simulink model "foc_blcd"  (R2022a)
settings: Solver=VariableStepAuto  StartTime=0.0  StopTime=1  RelTol=1e-3
values from neighbouring files (symbols this model uses):
  Idtarget = 0    [targetinitcoeffvalues.mat]
  Iqtarget = 10    [targetinitcoeffvalues.mat]
undefined symbols (not defined in the file or in its folder): deadTime_inv, f_spin
libraries: simulink x6, spsIdealSwitchLib x6, spsSeriesRLCBranchLib x4, spsMultimeterLib x3, slpidlib x2, spsAlphaBetaZerotoabcLib x1, spsAlphaBetaZerotodq0Lib x1, spsabctoAlphaBetaZeroLib x1, spsdq0toAlphaBetaZeroLib x1, spsDCVoltageSourceLib x1, spsGroundLib x1, spspowerguiLib x1
settings Model: Creator=1  LastModifiedBy=1
settings DebuggingCC: UnderSpecifiedDimensionMsg=warning

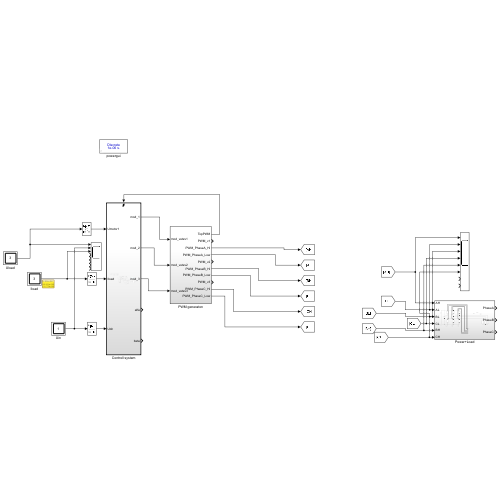
[thumbnail: Simulink's stored preview of the top-level diagram]
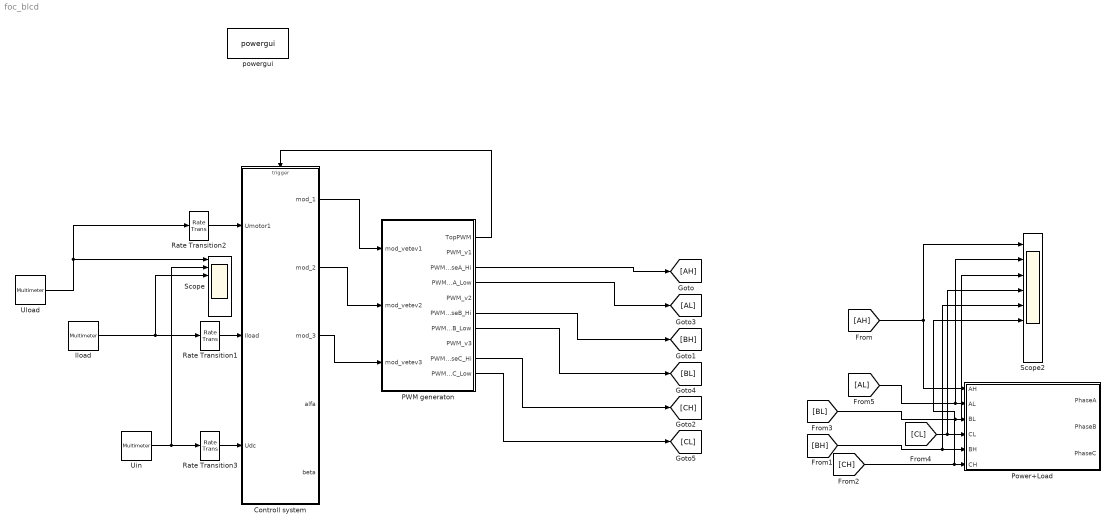
== system foc_blcd ==
  Controll system : Subsystem
  Iload : spsMultimeterLib/Multimeter  L=9  sel=[7 8 9]  yselected={}  Gain=[1 1 1]  OutputType=Complex  PlotAtSimulationStop=off  PhasorSimulation=off
  PWM generaton : Subsystem
  Power+Load : Subsystem
  Rate Transition1 : RateTransition  Integrity=off
  Rate Transition2 : RateTransition  Integrity=off
  Rate Transition3 : RateTransition  Integrity=off
  Scope : Scope  NumInputPorts=8
  Scope2 : Scope  NumInputPorts=8
  Uin : spsMultimeterLib/Multimeter  L=9  sel=1  yselected={}  Gain=1  OutputType=Complex  PlotAtSimulationStop=off  PhasorSimulation=off
  Uload : spsMultimeterLib/Multimeter  L=9  sel=[2 3 4]  yselected={}  Gain=[1 1 1]  OutputType=Complex  PlotAtSimulationStop=off  PhasorSimulation=off
  powergui : spspowerguiLib/powergui  Priority=1  SimulationMode=Discrete  SampleTime=1e-6  frequency=60  Iterations=50  frequencyindice=0  Pbase=100e6  ErrMax=1e-4  UnitsV=kV  UnitsW=MW  buscounter=0  FunctionMessages=off  echomessages=off  EnableUseOfTLC=off  CurrentSourceSwitches=off  DisableSnubberDevices=off  DisableRonSwitches=off  DisableVfSwitches=off  DisplayEquations=off  AutomaticDiscreteSolvers=off  SolverType=Tustin/Backward Euler (TBE)  Interpol=off  ExternalGateDelay=off  methode=off  Ts=100  x0status=blocks  SPID=on  SwTol=0  HookPort=off  NonlinearTolerance=1e-4  nMaxIteration=100  ContinueOnMaxIteration=off  RestoreLinks=warning  ResistiveCurrentMeasurement=off  Frange=[0:2:500]  Ylog=off  Xlog=on  ShowGrid=off  save=off  variable=ZData  structure=0  ZoomFFT=off  StartTime=0.0  cycles=1  DisplayStyle=1  fundamental=60  FreqAxis=off  MaxFrequency=1000  frequencyindicesteady=1  RmsSteady=1  display=off
  wires:
  Controll system/1(mod_1) -> PWM generaton/1(mod_vetev1)
  Controll system/2(mod_2) -> PWM generaton/2(mod_vetev2)
  Controll system/3(mod_3) -> PWM generaton/3(mod_vetev3)
  PWM generaton/1(TopPWM) -> Controll system/Trigger
  Uload/1 -> Rate Transition2/1, Scope/1
  Uin/1 -> Scope/2, Rate Transition3/1
  [AH] -> Scope2/1, Power+Load/1(AH)
  [CH] -> Scope2/6, Power+Load/6(CH)
  [BH] -> Power+Load/5(BH), Scope2/5
  [BL] -> Scope2/3, Power+Load/3(BL)
  [CL] -> Scope2/4, Power+Load/4(CL)
  [AL] -> Scope2/2, Power+Load/2(AL)
  PWM generaton/3(PWM_PhaseA_Hi) -> [AH]
  PWM generaton/4(PWM_PhaseA_Low) -> [AL]
  PWM generaton/6(PWM_PhaseB_Hi) -> [BH]
  PWM generaton/7(PWM_PhaseB_Low) -> [BL]
  PWM generaton/10(PWM_PhaseC_Low) -> [CL]
  PWM generaton/9(PWM_PhaseC_Hi) -> [CH]
  Iload/1 -> Scope/3, Rate Transition1/1
  Rate Transition2/1 -> Controll system/1(Umotor1)
  Rate Transition1/1 -> Controll system/2(Iload)
  Rate Transition3/1 -> Controll system/3(Udc)

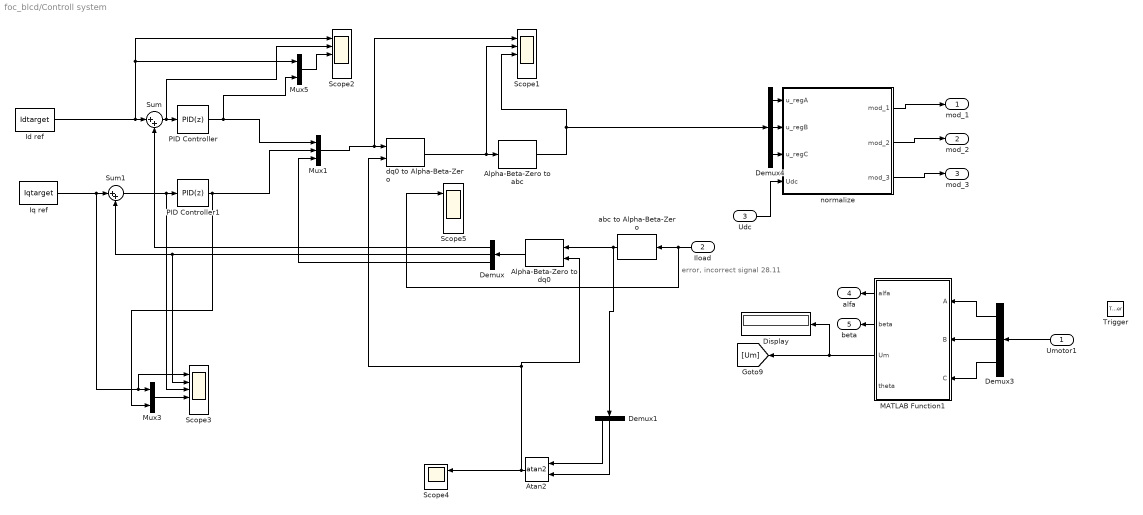
== system foc_blcd/Controll system ==
  note: error, incorrect signal 28.11
  Umotor1 : Inport
  Iload : Inport  Port=2
  Udc : Inport  Port=3
  Trigger : TriggerPort  VariantControl=(inherit)  PortDimensions=1
  Alpha-Beta-Zero to abc : spsAlphaBetaZerotoabcLib/Alpha-Beta-Zero to abc
      settings: SourceProductBaseCode=PS
  Alpha-Beta-Zero to dq0 : spsAlphaBetaZerotodq0Lib/Alpha-Beta-Zero to dq0  Alignment=90 degrees behind phase A axis
      settings: SourceProductBaseCode=PS
  Atan2 : Trigonometry  Operator=atan2
  Demux{,1,3..4} (4 alike) : Demux  Outputs=3
  Display : Display
  Id ref : Constant  Value=Idtarget
  Iq ref : Constant  Value=Iqtarget
  MATLAB Function1 : MATLAB Function  TreatAsAtomicUnit=on
  Mux1 : Mux  Inputs=3
  Mux3 : Mux  Inputs=2
  Mux5 : Mux  Inputs=2
  PID Controller : slpidlib/PID Controller  Controller=PID  Form=Parallel  TimeDomain=Discrete-time  UseExternalTs=off  SampleTime=-1  IntegratorMethod=Forward Euler  FilterMethod=Forward Euler  ControllerParametersSource=internal  P=1  I=0  UseKiTs=off  D=0  N=100  UseFilter=on  TunerSelectOption=Transfer Function Based (PID Tuner App)  InitialConditionSource=internal  InitialConditionForIntegrator=0  InitialConditionForFilter=0  DifferentiatorICPrevScaledInput=0  ExternalReset=none  TrackingMode=off  Kt=1  LimitOutput=off  SatLimitsSource=internal  UpperSaturationLimit=inf  LowerSaturationLimit=-inf  LinearizeAsGain=on  AntiWindupMode=none  Kb=1  POutMin=[]  POutMax=[]  IOutMin=[]  IOutMax=[]  DOutMin=[]  DOutMax=[]  NOutMin=[]  NOutMax=[]  SumOutMin=[]  SumOutMax=[]  SaturationOutMin=[]  SaturationOutMax=[]  PParamMin=[]  PParamMax=[]  IParamMin=[]  IParamMax=[]  DParamMin=[]  DParamMax=[]  NParamMin=[]  NParamMax=[]  KbParamMin=[]  KbParamMax=[]  KtParamMin=[]  KtParamMax=[]  KbOutMin=[]  KbOutMax=[]  KtOutMin=[]  KtOutMax=[]  IntegratorOutMin=[]  IntegratorOutMax=[]  FilterOutMin=[]  FilterOutMax=[]  SumI1OutMin=[]  SumI1OutMax=[]  SumI2OutMin=[]  SumI2OutMax=[]  SumI3OutMin=[]  SumI3OutMax=[]  SumI4OutMin=[]  SumI4OutMax=[]  SumDOutMin=[]  SumDOutMax=[]  DifferentiatorOutMin=[]  DifferentiatorOutMax=[]  FilterDiffOutCoefMin=[]  FilterDiffOutCoefMax=[]  ReciprocalOutMin=[]  ReciprocalOutMax=[]  SumDenOutMin=[]  SumDenOutMax=[]  SumNumOutMin=[]  SumNumOutMax=[]  DivideOutMin=[]  DivideOutMax=[]  UdiffTsProdOutMin=[]  UdiffTsProdOutMax=[]  NTsProdOutMin=[]  NTsProdOutMax=[]  UintegralTsProdOutMin=[]  UintegralTsProdOutMax=[]  UngainTsProdOutMin=[]  UngainTsProdOutMax=[]  IntegratorContinuousStateAttributes=''  IntegratorStateMustResolveToSignalObject=off  IntegratorRTWStateStorageClass=Auto  FilterContinuousStateAttributes=''  FilterStateMustResolveToSignalObject=off  FilterRTWStateStorageClass=Auto  ParallelPVariant=InternalParameters  IdealPVariant=Disabled  IVariant=InternalParameters  DVariant=InternalParameters  IntegratorVariant=Discrete  SatVariant=Disabled  AWVariant=Passthrough  PCopyVariant=Disabled  TRVariant=Disabled  FdbkBlocksVariant=Forward  IdealPFdbkVariant=Disabled  SatFdbkVariant=Disabled  DerivativeFilterVariant=ForwardEulerFilter  NVariant=InternalParameters  NCopyVariant=Disabled  FilterICVariant=InternalICsFilter  IntegratorICVariant=InternalICs  ExternalResetVariant=Disabled  TRSumVariant=Passthrough  SumFdbkVariant=Disabled  SumVariant=Sum_PID  TsampFilterVariant=InternalTs  TsampNgainVariant=Passthrough  TsampIntegralVariant=Passthrough  ExternalSaturationOutDataTypeStr=Inherit: Same as second input  aMode=0
  PID Controller1 : slpidlib/PID Controller  Controller=PID  Form=Parallel  TimeDomain=Discrete-time  UseExternalTs=off  SampleTime=-1  IntegratorMethod=Forward Euler  FilterMethod=Forward Euler  ControllerParametersSource=internal  P=1  I=0  UseKiTs=off  D=0  N=100  UseFilter=on  TunerSelectOption=Transfer Function Based (PID Tuner App)  InitialConditionSource=internal  InitialConditionForIntegrator=0  InitialConditionForFilter=0  DifferentiatorICPrevScaledInput=0  ExternalReset=none  TrackingMode=off  Kt=1  LimitOutput=off  SatLimitsSource=internal  UpperSaturationLimit=inf  LowerSaturationLimit=-inf  LinearizeAsGain=on  AntiWindupMode=none  Kb=1  POutMin=[]  POutMax=[]  IOutMin=[]  IOutMax=[]  DOutMin=[]  DOutMax=[]  NOutMin=[]  NOutMax=[]  SumOutMin=[]  SumOutMax=[]  SaturationOutMin=[]  SaturationOutMax=[]  PParamMin=[]  PParamMax=[]  IParamMin=[]  IParamMax=[]  DParamMin=[]  DParamMax=[]  NParamMin=[]  NParamMax=[]  KbParamMin=[]  KbParamMax=[]  KtParamMin=[]  KtParamMax=[]  KbOutMin=[]  KbOutMax=[]  KtOutMin=[]  KtOutMax=[]  IntegratorOutMin=[]  IntegratorOutMax=[]  FilterOutMin=[]  FilterOutMax=[]  SumI1OutMin=[]  SumI1OutMax=[]  SumI2OutMin=[]  SumI2OutMax=[]  SumI3OutMin=[]  SumI3OutMax=[]  SumI4OutMin=[]  SumI4OutMax=[]  SumDOutMin=[]  SumDOutMax=[]  DifferentiatorOutMin=[]  DifferentiatorOutMax=[]  FilterDiffOutCoefMin=[]  FilterDiffOutCoefMax=[]  ReciprocalOutMin=[]  ReciprocalOutMax=[]  SumDenOutMin=[]  SumDenOutMax=[]  SumNumOutMin=[]  SumNumOutMax=[]  DivideOutMin=[]  DivideOutMax=[]  UdiffTsProdOutMin=[]  UdiffTsProdOutMax=[]  NTsProdOutMin=[]  NTsProdOutMax=[]  UintegralTsProdOutMin=[]  UintegralTsProdOutMax=[]  UngainTsProdOutMin=[]  UngainTsProdOutMax=[]  IntegratorContinuousStateAttributes=''  IntegratorStateMustResolveToSignalObject=off  IntegratorRTWStateStorageClass=Auto  FilterContinuousStateAttributes=''  FilterStateMustResolveToSignalObject=off  FilterRTWStateStorageClass=Auto  ParallelPVariant=InternalParameters  IdealPVariant=Disabled  IVariant=InternalParameters  DVariant=InternalParameters  IntegratorVariant=Discrete  SatVariant=Disabled  AWVariant=Passthrough  PCopyVariant=Disabled  TRVariant=Disabled  FdbkBlocksVariant=Forward  IdealPFdbkVariant=Disabled  SatFdbkVariant=Disabled  DerivativeFilterVariant=ForwardEulerFilter  NVariant=InternalParameters  NCopyVariant=Disabled  FilterICVariant=InternalICsFilter  IntegratorICVariant=InternalICs  ExternalResetVariant=Disabled  TRSumVariant=Passthrough  SumFdbkVariant=Disabled  SumVariant=Sum_PID  TsampFilterVariant=InternalTs  TsampNgainVariant=Passthrough  TsampIntegralVariant=Passthrough  ExternalSaturationOutDataTypeStr=Inherit: Same as second input  aMode=0
  Scope{1..3,5} (4 alike) : Scope  NumInputPorts=5
  Scope4 : Scope  NumInputPorts=2
  Sum : Sum  Inputs=|++
  Sum1 : Sum  Inputs=|++
  abc to Alpha-Beta-Zero : spsabctoAlphaBetaZeroLib/abc to Alpha-Beta-Zero
      settings: SourceProductBaseCode=PS
  dq0 to Alpha-Beta-Zero : spsdq0toAlphaBetaZeroLib/dq0 to Alpha-Beta-Zero  Alignment=90 degrees behind phase A axis
      settings: SourceProductBaseCode=PS
  normalize : MATLAB Function  TreatAsAtomicUnit=on
  mod_1 : Outport
  mod_2 : Outport  Port=2
  mod_3 : Outport  Port=3
  alfa : Outport  Port=4
  beta : Outport  Port=5
  wires:
  abc to Alpha-Beta-Zero/1 -> Demux1/1, Alpha-Beta-Zero to dq0/1
  Demux4/3 -> normalize/3(u_regC)
  Id ref/1 -> Mux5/1, Scope2/1, Sum/1
  MATLAB Function1/3(Um) -> [Um], Display/1
  Demux/1 -> Sum/2
  Sum1/1 -> Scope3/3, PID Controller1/1
  Alpha-Beta-Zero to abc/1 -> Scope1/3, Demux4/1
  Mux1/1 -> Scope1/1, dq0 to Alpha-Beta-Zero/1
  Demux/2 -> Sum1/2, Scope3/2
  Demux4/1 -> normalize/1(u_regA)
  Iq ref/1 -> Scope3/1, Mux3/1, Sum1/1
  dq0 to Alpha-Beta-Zero/1 -> Scope1/2, Alpha-Beta-Zero to abc/1
  Sum/1 -> Scope2/2, PID Controller/1
  Demux3/1 -> MATLAB Function1/1(A)
  Demux/3 -> Mux1/3
  PID Controller/1 -> Mux1/1, Mux5/2
  Demux4/2 -> normalize/2(u_regB)
  Alpha-Beta-Zero to dq0/1 -> Demux/1
  PID Controller1/1 -> Mux1/2, Mux3/2
  Demux3/3 -> MATLAB Function1/3(C)
  Demux3/2 -> MATLAB Function1/2(B)
  normalize/2(mod_2) -> mod_2/1
  MATLAB Function1/2(beta) -> beta/1
  MATLAB Function1/1(alfa) -> alfa/1
  normalize/3(mod_3) -> mod_3/1
  normalize/1(mod_1) -> mod_1/1
  Umotor1/1 -> Demux3/1
  Iload/1 -> abc to Alpha-Beta-Zero/1, Scope5/1
  Udc/1 -> normalize/4(Udc)
  Atan2/1 -> Alpha-Beta-Zero to dq0/2, dq0 to Alpha-Beta-Zero/2, Scope4/1
  Demux1/1 -> Atan2/1
  Demux1/2 -> Atan2/2
  Mux3/1 -> Scope3/4
  Mux5/1 -> Scope2/3

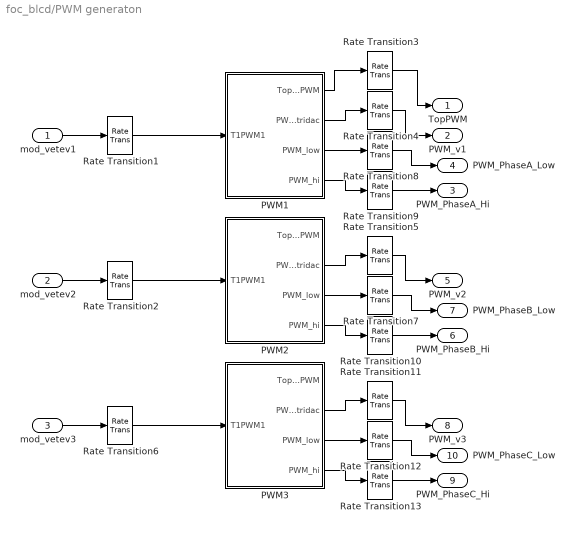
== system foc_blcd/PWM generaton ==
  mod_vetev1 : Inport
  mod_vetev2 : Inport  Port=2
  mod_vetev3 : Inport  Port=3
  PWM1 : Subsystem
  PWM2 : Subsystem
  PWM3 : Subsystem
  Rate Transition{1..13} (13 alike) : RateTransition  Integrity=off
  TopPWM : Outport
  PWM_v1 : Outport  Port=2
  PWM_PhaseA_Hi : Outport  Port=3
  PWM_PhaseA_Low : Outport  Port=4
  PWM_v2 : Outport  Port=5
  PWM_PhaseB_Hi : Outport  Port=6
  PWM_PhaseB_Low : Outport  Port=7
  PWM_v3 : Outport  Port=8
  PWM_PhaseC_Hi : Outport  Port=9
  PWM_PhaseC_Low : Outport  Port=10
  wires:
  mod_vetev1/1 -> Rate Transition1/1
  mod_vetev2/1 -> Rate Transition2/1
  PWM1/2(PWM_stridac) -> Rate Transition4/1
  Rate Transition1/1 -> PWM1/1(T1PWM1)
  Rate Transition2/1 -> PWM2/1(T1PWM1)
  Rate Transition4/1 -> PWM_v1/1
  Rate Transition3/1 -> TopPWM/1
  PWM1/1(TopBot_PWM) -> Rate Transition3/1
  Rate Transition6/1 -> PWM3/1(T1PWM1)
  mod_vetev3/1 -> Rate Transition6/1
  PWM1/3(PWM_low) -> Rate Transition8/1
  PWM1/4(PWM_hi) -> Rate Transition9/1
  Rate Transition9/1 -> PWM_PhaseA_Hi/1
  Rate Transition8/1 -> PWM_PhaseA_Low/1
  Rate Transition10/1 -> PWM_PhaseB_Hi/1
  Rate Transition7/1 -> PWM_PhaseB_Low/1
  Rate Transition5/1 -> PWM_v2/1
  PWM2/4(PWM_hi) -> Rate Transition10/1
  PWM2/2(PWM_stridac) -> Rate Transition5/1
  PWM2/3(PWM_low) -> Rate Transition7/1
  Rate Transition13/1 -> PWM_PhaseC_Hi/1
  Rate Transition12/1 -> PWM_PhaseC_Low/1
  Rate Transition11/1 -> PWM_v3/1
  PWM3/4(PWM_hi) -> Rate Transition13/1
  PWM3/2(PWM_stridac) -> Rate Transition11/1
  PWM3/3(PWM_low) -> Rate Transition12/1

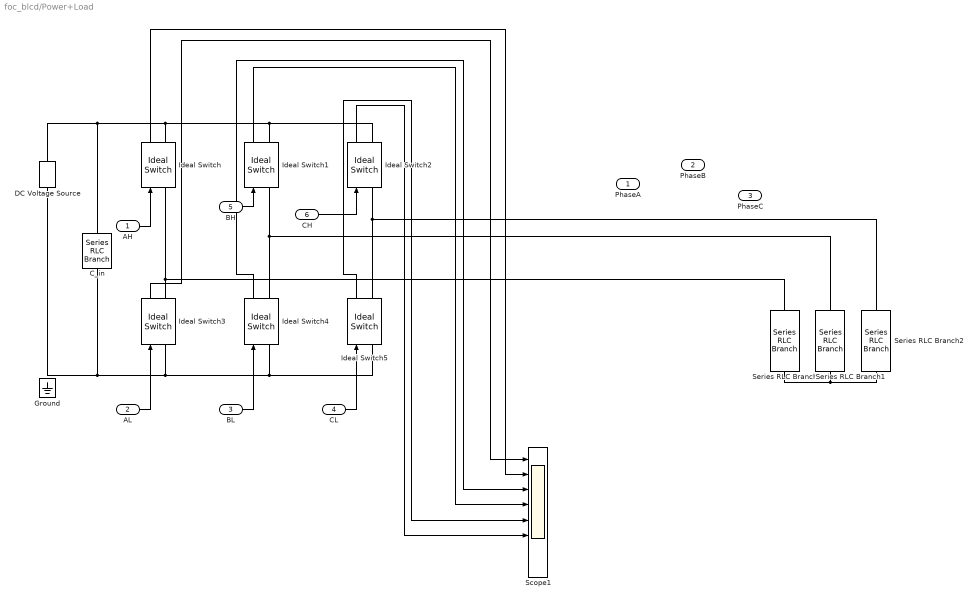
== system foc_blcd/Power+Load ==
  AH : Inport
  AL : Inport  Port=2
  BL : Inport  Port=3
  CL : Inport  Port=4
  BH : Inport  Port=5
  CH : Inport  Port=6
  C_in : spsSeriesRLCBranchLib/Series RLC Branch  LConnTagsString=__new0  RConnTagsString=__new0  BranchType=RC  Resistance=1e-6  Inductance=0  SetiL0=off  InitialCurrent=0  Capacitance=1e-4  Setx0=off  InitialVoltage=0  Measurements=Branch voltage and current
  DC Voltage Source : spsDCVoltageSourceLib/DC Voltage Source  Amplitude=48  Measurements=Voltage
  Ground : spsGroundLib/Ground  LConnTagsString=a
  Ideal Switch{,1..5} (6 alike) : spsIdealSwitchLib/Ideal Switch  Ron=0.001  Lon=0  IC=0  Rs=1e5  Cs=inf  Measurements=on
  Scope1 : Scope  NumInputPorts=8
  Series RLC Branch : spsSeriesRLCBranchLib/Series RLC Branch  LConnTagsString=__new0  RConnTagsString=__new0  BranchType=RLC  Resistance=1  Inductance=1e-6  SetiL0=off  InitialCurrent=0  Capacitance=0  Setx0=off  InitialVoltage=0  Measurements=Branch voltage and current
  Series RLC Branch1 : spsSeriesRLCBranchLib/Series RLC Branch  LConnTagsString=__new0  RConnTagsString=__new0  BranchType=RLC  Resistance=1  Inductance=1e-6  SetiL0=off  InitialCurrent=0  Capacitance=0  Setx0=off  InitialVoltage=0  Measurements=Branch voltage and current
  Series RLC Branch2 : spsSeriesRLCBranchLib/Series RLC Branch  LConnTagsString=__new0  RConnTagsString=__new0  BranchType=RLC  Resistance=1  Inductance=1e-6  SetiL0=off  InitialCurrent=0  Capacitance=0  Setx0=off  InitialVoltage=0  Measurements=Branch voltage and current
  PhaseA : Outport
  PhaseB : Outport  Port=2
  PhaseC : Outport  Port=3
  wires:
  AH/1 -> Ideal Switch/1
  Ideal Switch4/1 -> Scope1/3
  CL/1 -> Ideal Switch5/1
  Ideal Switch2/1 -> Scope1/6
  BL/1 -> Ideal Switch4/1
  BH/1 -> Ideal Switch1/1
  Ideal Switch3/1 -> Scope1/1
  Ideal Switch1/1 -> Scope1/4
  Ideal Switch/1 -> Scope1/2
  AL/1 -> Ideal Switch3/1
  Ideal Switch5/1 -> Scope1/5
  CH/1 -> Ideal Switch2/1
  connections:
  Ideal Switch2/RConn1 -- C_in/LConn1 -- DC Voltage Source/RConn1 -- Ideal Switch/RConn1 -- Ideal Switch1/RConn1
  Ideal Switch3/RConn1 -- Ideal Switch/LConn1 -- Series RLC Branch/LConn1
  DC Voltage Source/LConn1 -- C_in/RConn1 -- Ideal Switch3/LConn1 -- Ideal Switch4/LConn1 -- Ideal Switch5/LConn1
  Ideal Switch2/LConn1 -- Series RLC Branch2/LConn1 -- Ideal Switch5/RConn1
  Ideal Switch4/RConn1 -- Series RLC Branch1/LConn1 -- Ideal Switch1/LConn1
  Series RLC Branch/RConn1 -- Series RLC Branch1/RConn1 -- Series RLC Branch2/RConn1

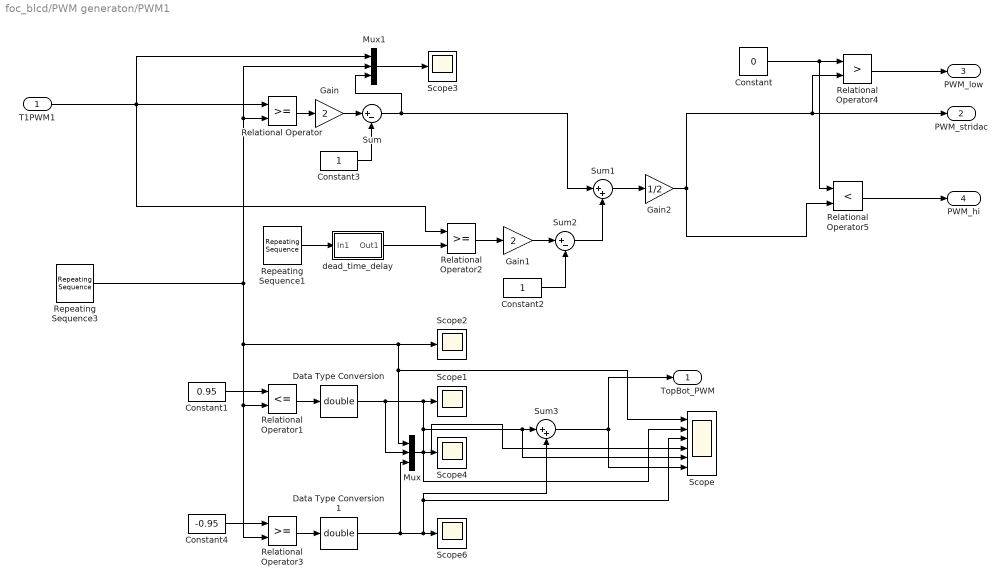
== system foc_blcd/PWM generaton/PWM1 ==
  T1PWM1 : Inport
  Constant : Constant  Value=0
  Constant1 : Constant  Value=0.95
  Constant2 : Constant
  Constant3 : Constant
  Constant4 : Constant  Value=-0.95
  Data Type Conversion : DataTypeConversion  OutDataTypeStr=double  SaturateOnIntegerOverflow=off  RndMeth=Floor
  Data Type Conversion1 : DataTypeConversion  OutDataTypeStr=double  SaturateOnIntegerOverflow=off  RndMeth=Floor
  Gain : Gain  Gain=2
  Gain1 : Gain  Gain=2
  Gain2 : Gain  Gain=1/2
  Mux : Mux  Inputs=3
  Mux1 : Mux  Inputs=3
  Relational Operator : RelationalOperator  OutDataTypeStr=boolean  InputSameDT=off
  Relational Operator1 : RelationalOperator  Operator=<=  OutDataTypeStr=boolean  InputSameDT=off
  Relational Operator2 : RelationalOperator  OutDataTypeStr=boolean  InputSameDT=off
  Relational Operator3 : RelationalOperator  OutDataTypeStr=boolean  InputSameDT=off
  Relational Operator4 : RelationalOperator  Operator=>  OutDataTypeStr=boolean  InputSameDT=off
  Relational Operator5 : RelationalOperator  Operator=<  OutDataTypeStr=boolean  InputSameDT=off
  Repeating Sequence1 : simulink/Sources/Repeating Sequence  rep_seq_t=[0 1/(2*f_spin) 1/f_spin]  rep_seq_y=[-1 1 -1]
  Repeating Sequence3 : simulink/Sources/Repeating Sequence  rep_seq_t=[0 1/(2*f_spin) 1/f_spin]  rep_seq_y=[-1 1 -1]
  Scope : Scope  NumInputPorts=6
  Scope{1..4,6} (5 alike) : Scope
  Sum : Sum  Inputs=|+-
  Sum1 : Sum  Inputs=|++
  Sum2 : Sum  Inputs=|+-
  Sum3 : Sum  Inputs=|++
  dead_time_delay : Subsystem
  TopBot_PWM : Outport
  PWM_stridac : Outport  Port=2
  PWM_low : Outport  Port=3
  PWM_hi : Outport  Port=4
  wires:
  Relational Operator/1 -> Gain/1
  Gain/1 -> Sum/1
  Constant3/1 -> Sum/2
  Constant1/1 -> Relational Operator1/1
  Relational Operator1/1 -> Data Type Conversion/1
  Mux/1 -> Scope/4, Scope4/1
  Sum/1 -> Sum1/1, Mux1/3
  Data Type Conversion/1 -> Mux/2, Scope/5, Sum3/1, Scope/2, Scope1/1
  Mux1/1 -> Scope3/1
  T1PWM1/1 -> Relational Operator2/1, Mux1/1, Relational Operator/1
  Repeating Sequence1/1 -> dead_time_delay/1(In1)
  dead_time_delay/1(Out1) -> Relational Operator2/2
  Relational Operator2/1 -> Gain1/1
  Sum1/1 -> Gain2/1
  Gain1/1 -> Sum2/1
  Sum2/1 -> Sum1/2
  Constant2/1 -> Sum2/2
  Gain2/1 -> PWM_stridac/1, Relational Operator4/2, Relational Operator5/2
  Repeating Sequence3/1 -> Mux1/2, Relational Operator/2, Mux/1, Scope/1, Scope2/1, Relational Operator3/2, Relational Operator1/2
  Constant4/1 -> Relational Operator3/1
  Relational Operator3/1 -> Data Type Conversion1/1
  Data Type Conversion1/1 -> Mux/3, Sum3/2, Scope/3, Scope6/1
  Sum3/1 -> Scope/6, TopBot_PWM/1
  Constant/1 -> Relational Operator5/1, Relational Operator4/1
  Relational Operator4/1 -> PWM_low/1
  Relational Operator5/1 -> PWM_hi/1

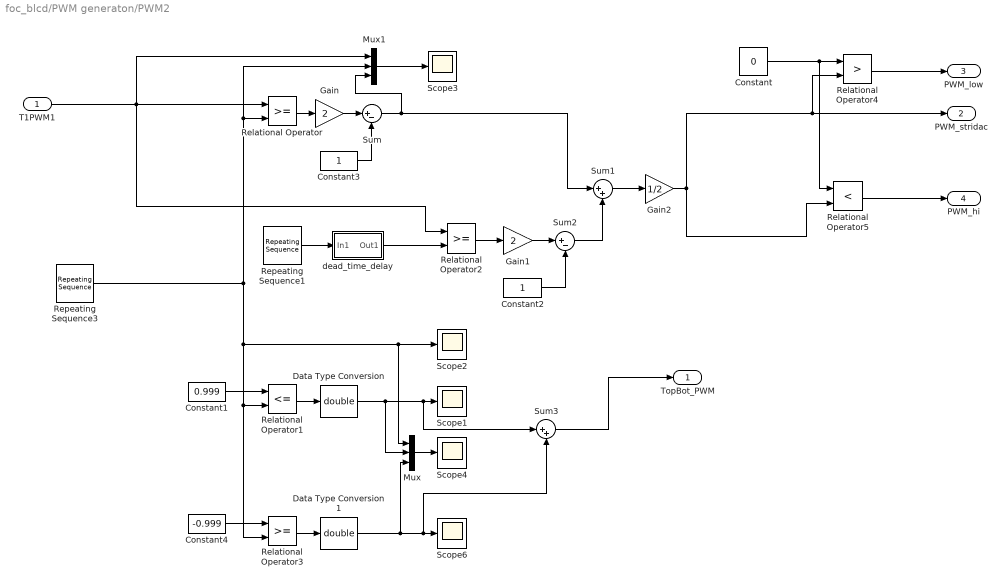
== system foc_blcd/PWM generaton/PWM2 ==
  T1PWM1 : Inport
  Constant : Constant  Value=0
  Constant1 : Constant  Value=0.999
  Constant2 : Constant
  Constant3 : Constant
  Constant4 : Constant  Value=-0.999
  Data Type Conversion : DataTypeConversion  OutDataTypeStr=double  SaturateOnIntegerOverflow=off  RndMeth=Floor
  Data Type Conversion1 : DataTypeConversion  OutDataTypeStr=double  SaturateOnIntegerOverflow=off  RndMeth=Floor
  Gain : Gain  Gain=2
  Gain1 : Gain  Gain=2
  Gain2 : Gain  Gain=1/2
  Mux : Mux  Inputs=3
  Mux1 : Mux  Inputs=3
  Relational Operator : RelationalOperator  OutDataTypeStr=boolean  InputSameDT=off
  Relational Operator1 : RelationalOperator  Operator=<=  OutDataTypeStr=boolean  InputSameDT=off
  Relational Operator2 : RelationalOperator  OutDataTypeStr=boolean  InputSameDT=off
  Relational Operator3 : RelationalOperator  OutDataTypeStr=boolean  InputSameDT=off
  Relational Operator4 : RelationalOperator  Operator=>  OutDataTypeStr=boolean  InputSameDT=off
  Relational Operator5 : RelationalOperator  Operator=<  OutDataTypeStr=boolean  InputSameDT=off
  Repeating Sequence1 : simulink/Sources/Repeating Sequence  rep_seq_t=[0 1/(2*f_spin) 1/f_spin]  rep_seq_y=[-1 1 -1]
  Repeating Sequence3 : simulink/Sources/Repeating Sequence  rep_seq_t=[0 1/(2*f_spin) 1/f_spin]  rep_seq_y=[-1 1 -1]
  Scope{1..4,6} (5 alike) : Scope
  Sum : Sum  Inputs=|+-
  Sum1 : Sum  Inputs=|++
  Sum2 : Sum  Inputs=|+-
  Sum3 : Sum  Inputs=|++
  dead_time_delay : Subsystem
  TopBot_PWM : Outport
  PWM_stridac : Outport  Port=2
  PWM_low : Outport  Port=3
  PWM_hi : Outport  Port=4
  wires:
  Relational Operator/1 -> Gain/1
  Gain/1 -> Sum/1
  Constant3/1 -> Sum/2
  Constant1/1 -> Relational Operator1/1
  Relational Operator1/1 -> Data Type Conversion/1
  Mux/1 -> Scope4/1
  Sum/1 -> Sum1/1, Mux1/3
  Data Type Conversion/1 -> Mux/2, Sum3/1, Scope1/1
  Mux1/1 -> Scope3/1
  T1PWM1/1 -> Relational Operator2/1, Mux1/1, Relational Operator/1
  Repeating Sequence1/1 -> dead_time_delay/1(In1)
  dead_time_delay/1(Out1) -> Relational Operator2/2
  Relational Operator2/1 -> Gain1/1
  Sum1/1 -> Gain2/1
  Gain1/1 -> Sum2/1
  Sum2/1 -> Sum1/2
  Constant2/1 -> Sum2/2
  Gain2/1 -> PWM_stridac/1, Relational Operator4/2, Relational Operator5/2
  Repeating Sequence3/1 -> Mux1/2, Relational Operator/2, Mux/1, Scope2/1, Relational Operator3/2, Relational Operator1/2
  Constant4/1 -> Relational Operator3/1
  Relational Operator3/1 -> Data Type Conversion1/1
  Data Type Conversion1/1 -> Mux/3, Sum3/2, Scope6/1
  Sum3/1 -> TopBot_PWM/1
  Constant/1 -> Relational Operator5/1, Relational Operator4/1
  Relational Operator4/1 -> PWM_low/1
  Relational Operator5/1 -> PWM_hi/1

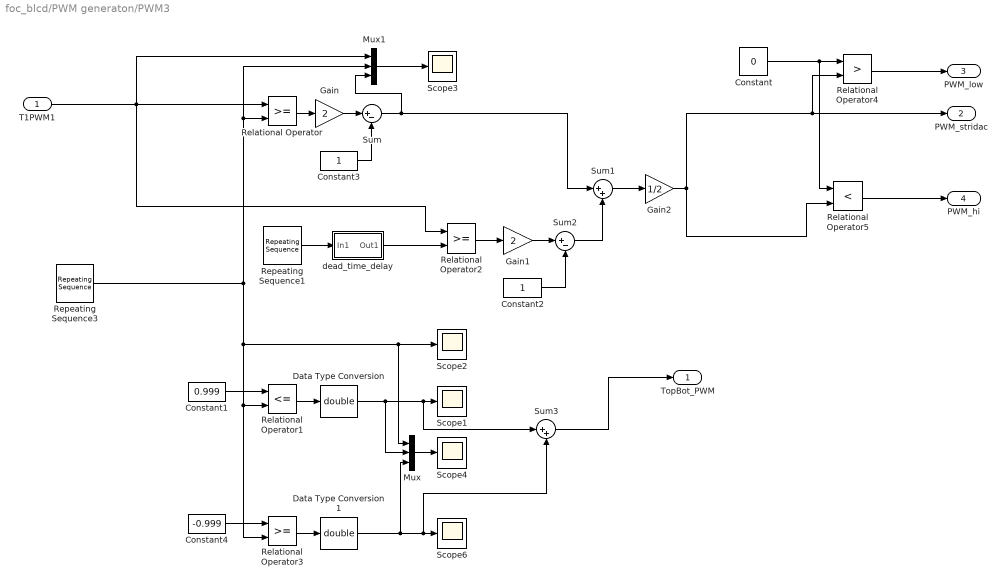
== system foc_blcd/PWM generaton/PWM3 ==
  T1PWM1 : Inport
  Constant : Constant  Value=0
  Constant1 : Constant  Value=0.999
  Constant2 : Constant
  Constant3 : Constant
  Constant4 : Constant  Value=-0.999
  Data Type Conversion : DataTypeConversion  OutDataTypeStr=double  SaturateOnIntegerOverflow=off  RndMeth=Floor
  Data Type Conversion1 : DataTypeConversion  OutDataTypeStr=double  SaturateOnIntegerOverflow=off  RndMeth=Floor
  Gain : Gain  Gain=2
  Gain1 : Gain  Gain=2
  Gain2 : Gain  Gain=1/2
  Mux : Mux  Inputs=3
  Mux1 : Mux  Inputs=3
  Relational Operator : RelationalOperator  OutDataTypeStr=boolean  InputSameDT=off
  Relational Operator1 : RelationalOperator  Operator=<=  OutDataTypeStr=boolean  InputSameDT=off
  Relational Operator2 : RelationalOperator  OutDataTypeStr=boolean  InputSameDT=off
  Relational Operator3 : RelationalOperator  OutDataTypeStr=boolean  InputSameDT=off
  Relational Operator4 : RelationalOperator  Operator=>  OutDataTypeStr=boolean  InputSameDT=off
  Relational Operator5 : RelationalOperator  Operator=<  OutDataTypeStr=boolean  InputSameDT=off
  Repeating Sequence1 : simulink/Sources/Repeating Sequence  rep_seq_t=[0 1/(2*f_spin) 1/f_spin]  rep_seq_y=[-1 1 -1]
  Repeating Sequence3 : simulink/Sources/Repeating Sequence  rep_seq_t=[0 1/(2*f_spin) 1/f_spin]  rep_seq_y=[-1 1 -1]
  Scope{1..4,6} (5 alike) : Scope
  Sum : Sum  Inputs=|+-
  Sum1 : Sum  Inputs=|++
  Sum2 : Sum  Inputs=|+-
  Sum3 : Sum  Inputs=|++
  dead_time_delay : Subsystem
  TopBot_PWM : Outport
  PWM_stridac : Outport  Port=2
  PWM_low : Outport  Port=3
  PWM_hi : Outport  Port=4
  wires:
  Relational Operator/1 -> Gain/1
  Gain/1 -> Sum/1
  Constant3/1 -> Sum/2
  Constant1/1 -> Relational Operator1/1
  Relational Operator1/1 -> Data Type Conversion/1
  Mux/1 -> Scope4/1
  Sum/1 -> Sum1/1, Mux1/3
  Data Type Conversion/1 -> Mux/2, Sum3/1, Scope1/1
  Mux1/1 -> Scope3/1
  T1PWM1/1 -> Relational Operator2/1, Mux1/1, Relational Operator/1
  Repeating Sequence1/1 -> dead_time_delay/1(In1)
  dead_time_delay/1(Out1) -> Relational Operator2/2
  Relational Operator2/1 -> Gain1/1
  Sum1/1 -> Gain2/1
  Gain1/1 -> Sum2/1
  Sum2/1 -> Sum1/2
  Constant2/1 -> Sum2/2
  Gain2/1 -> PWM_stridac/1, Relational Operator4/2, Relational Operator5/2
  Repeating Sequence3/1 -> Mux1/2, Relational Operator/2, Mux/1, Scope2/1, Relational Operator3/2, Relational Operator1/2
  Constant4/1 -> Relational Operator3/1
  Relational Operator3/1 -> Data Type Conversion1/1
  Data Type Conversion1/1 -> Mux/3, Sum3/2, Scope6/1
  Sum3/1 -> TopBot_PWM/1
  Constant/1 -> Relational Operator5/1, Relational Operator4/1
  Relational Operator4/1 -> PWM_low/1
  Relational Operator5/1 -> PWM_hi/1

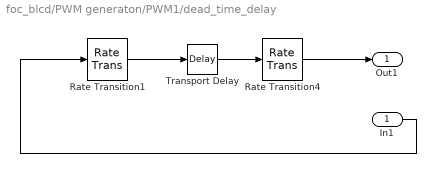
== system foc_blcd/PWM generaton/PWM1/dead_time_delay ==
  In1 : Inport
  Rate Transition1 : RateTransition  Integrity=off
  Rate Transition4 : RateTransition  Integrity=off
  Transport Delay : TransportDelay  DelayTime=deadTime_inv
  Out1 : Outport
  wires:
  In1/1 -> Rate Transition1/1
  Rate Transition4/1 -> Out1/1
  Rate Transition1/1 -> Transport Delay/1
  Transport Delay/1 -> Rate Transition4/1

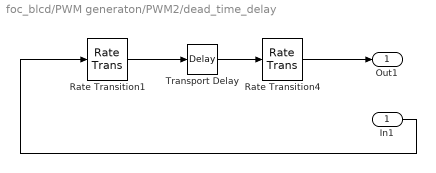
== system foc_blcd/PWM generaton/PWM2/dead_time_delay ==
  In1 : Inport
  Rate Transition1 : RateTransition  Integrity=off
  Rate Transition4 : RateTransition  Integrity=off
  Transport Delay : TransportDelay  DelayTime=deadTime_inv
  Out1 : Outport
  wires:
  In1/1 -> Rate Transition1/1
  Rate Transition4/1 -> Out1/1
  Rate Transition1/1 -> Transport Delay/1
  Transport Delay/1 -> Rate Transition4/1

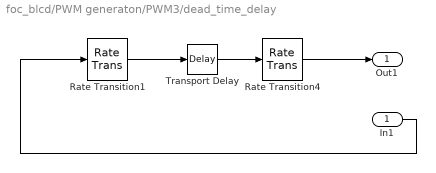
== system foc_blcd/PWM generaton/PWM3/dead_time_delay ==
  In1 : Inport
  Rate Transition1 : RateTransition  Integrity=off
  Rate Transition4 : RateTransition  Integrity=off
  Transport Delay : TransportDelay  DelayTime=deadTime_inv
  Out1 : Outport
  wires:
  In1/1 -> Rate Transition1/1
  Rate Transition4/1 -> Out1/1
  Rate Transition1/1 -> Transport Delay/1
  Transport Delay/1 -> Rate Transition4/1

== matlab function foc_blcd/Controll system/MATLAB Function1 ==
  data: A input; alfa output; B input; beta output; C input; Um output; theta output
function [alfa , beta, Um, theta] = fcn(A, B, C)

alfa = ((2/3)*(A-B/2-C/2))/1;
beta = ((2/3)*((sqrt(3)/2*B)-(sqrt(3)/2*C)))/1;

Um = sqrt(alfa*alfa + beta*beta);
theta = atan2(beta,alfa);

== matlab function foc_blcd/Controll system/normalize ==
  data: mod_1 output; mod_2 output; mod_3 output; u_regA input; u_regB input; u_regC input; Udc input
function [mod_1,mod_2,mod_3]  = normalize(u_regA,u_regB,u_regC,Udc)


mod_1=u_regA/Udc;
mod_2=u_regB/Udc;
mod_3=u_regC/Udc;
